simulink model "OnePhInverterCS_17b"  (R2020a)
settings: Solver=ode23tb  StartTime=0.0  StopTime=1  MaxStep=1e-3  RelTol=1e-3
libraries: powerlib x13, powerlib_meascontrol x10
settings Model: Creator=theo  LastModifiedBy=Theodore
settings DebuggingCC: ArithmeticOperatorsInVariantConditions=warning
settings SFSimCC: CustomCodeUndefinedFunction=UseInterfaceOnly

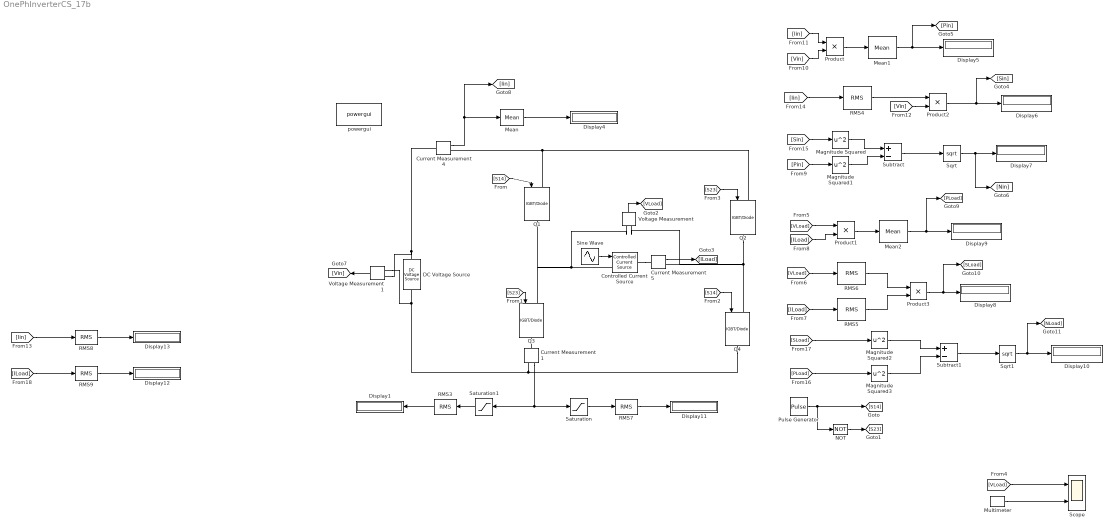
== system OnePhInverterCS_17b ==
  Controlled Current Source : powerlib/Electrical Sources/Controlled Current Source  Initialize=on  Source_Type=AC  Amplitude=10  Phase=0  Frequency=0  Measurements=Current
  Current Measurement1 : powerlib/Measurements/Current Measurement  PhasorSimulation=off  OutputType=Complex  PSBequivalent=0
  Current Measurement4 : powerlib/Measurements/Current Measurement  PhasorSimulation=off  OutputType=Complex  PSBequivalent=0
  Current Measurement5 : powerlib/Measurements/Current Measurement  PhasorSimulation=off  OutputType=Complex  PSBequivalent=0
  DC Voltage Source : powerlib/Electrical Sources/DC Voltage Source  Amplitude=537.97  Measurements=None
  Display{1,4..13} (11 alike) : Display
  Magnitude Squared{,1..3} (4 alike) : Math  Operator=square  SaturateOnIntegerOverflow=on
  Mean : powerlib_meascontrol/Measurements/Mean  Freq=50  Vinit=0  Ts=0
  Mean1 : powerlib_meascontrol/Measurements/Mean  Freq=50  Vinit=0  Ts=0
  Mean2 : powerlib_meascontrol/Measurements/Mean  Freq=50  Vinit=0  Ts=0
  Multimeter : powerlib/Measurements/Multimeter  PhasorSimulation=off  OutputType=Complex  sel=1  L=1  Gain=1  yselected={'Isrc: Controlled Current Source'};  PSBOutputType=1  PSBequivalent=0  AxesSetting=[0,0.1,-100,100]  Display=0  SavedBlockNames=-11
  NOT : Logic  Operator=NOT  IconShape=distinctive  AllPortsSameDT=off  OutDataTypeStr=boolean
  Product{,1..3} (4 alike) : Product
  Pulse Generator : DiscretePulseGenerator  PulseType=Time based  Period=0.02  PulseWidth=50
  Q{1..4} (4 alike) : powerlib/Power Electronics/IGBT//Diode  Ron=1e-3  Rs=1e5  Cs=inf  Measurements=off
  RMS{3..9} (7 alike) : powerlib_meascontrol/Measurements/RMS  TrueRMS=on  Freq=50  RMSInit=120  Ts=0
  Saturation : Saturate  UpperLimit=0  LowerLimit=-100
  Saturation1 : Saturate  UpperLimit=100  LowerLimit=0
  Scope : Scope  NumInputPorts=2
  Sine Wave : Sin  Amplitude=10  Frequency=2*pi*50  Phase=-pi/6  SampleTime=0
  Sqrt : Sqrt  SaturateOnIntegerOverflow=on
  Sqrt1 : Sqrt  SaturateOnIntegerOverflow=on
  Subtract : Sum  Inputs=+-
  Subtract1 : Sum  Inputs=+-
  Voltage Measurement : powerlib/Measurements/Voltage Measurement  PhasorSimulation=off  OutputType=Complex  PSBequivalent=0
  Voltage Measurement1 : powerlib/Measurements/Voltage Measurement  PhasorSimulation=off  OutputType=Complex  PSBequivalent=0
  powergui : powerlib/powergui  Priority=1  SimulationMode=Continuous  SampleTime=50e-6  frequency=60  Iterations=50  frequencyindice=0  Pbase=100e6  ErrMax=1e-4  UnitsV=kV  UnitsW=MW  buscounter=0  FunctionMessages=off  echomessages=off  EnableUseOfTLC=off  CurrentSourceSwitches=off  DisableSnubberDevices=on  DisableRonSwitches=on  DisableVfSwitches=on  DisplayEquations=off  AutomaticDiscreteSolvers=off  SolverType=Tustin/Backward Euler (TBE)  Interpol=off  ExternalGateDelay=off  methode=off  Ts=100  x0status=blocks  SPID=on  SwTol=0  HookPort=off  NonlinearTolerance=1e-4  nMaxIteration=100  ContinueOnMaxIteration=off  RestoreLinks=warning  ResistiveCurrentMeasurement=off  Frange=[0:2:500]  Ylog=off  Xlog=on  ShowGrid=off  save=off  variable=ZData  structure=0  ZoomFFT=off  StartTime=0.0  cycles=1  DisplayStyle=1  fundamental=60  FreqAxis=off  MaxFrequency=1000  frequencyindicesteady=1  RmsSteady=1  display=off
  wires:
  [S14] -> Q1/1
  NOT/1 -> [S23]
  Voltage Measurement/1 -> [VLoad]
  Multimeter/1 -> Scope/2
  [S14] -> Q4/1
  [S23] -> Q3/1
  [VLoad] -> Scope/1
  [S23] -> Q2/1
  Pulse Generator/1 -> NOT/1, [S14]
  Sine Wave/1 -> Controlled Current Source/1
  Current Measurement1/1 -> Saturation1/1, Saturation/1
  Mean/1 -> Display4/1
  [Pin] -> Magnitude Squared1/1
  [Iin] -> Product/1
  Magnitude Squared1/1 -> Subtract/2
  [Iin] -> RMS4/1
  RMS4/1 -> Product2/1
  Sqrt/1 -> [Nin], Display7/1
  [Sin] -> Magnitude Squared/1
  [Vin] -> Product2/2
  [Vin] -> Product/2
  Subtract/1 -> Sqrt/1
  Magnitude Squared/1 -> Subtract/1
  Product2/1 -> [Sin], Display6/1
  Mean1/1 -> [Pin], Display5/1
  Product/1 -> Mean1/1
  Product1/1 -> Mean2/1
  Sqrt1/1 -> [NLoad], Display10/1
  Product3/1 -> [SLoad], Display8/1
  [PLoad] -> Magnitude Squared3/1
  [SLoad] -> Magnitude Squared2/1
  Magnitude Squared2/1 -> Subtract1/1
  Magnitude Squared3/1 -> Subtract1/2
  [ILoad] -> RMS5/1
  RMS6/1 -> Product3/1
  [ILoad] -> Product1/2
  [VLoad] -> Product1/1
  Subtract1/1 -> Sqrt1/1
  Mean2/1 -> [PLoad], Display9/1
  RMS5/1 -> Product3/2
  [VLoad] -> RMS6/1
  Current Measurement4/1 -> [Iin], Mean/1
  Voltage Measurement1/1 -> [Vin]
  Current Measurement5/1 -> [ILoad]
  Saturation/1 -> RMS7/1
  RMS7/1 -> Display11/1
  RMS3/1 -> Display1/1
  Saturation1/1 -> RMS3/1
  RMS8/1 -> Display13/1
  RMS9/1 -> Display12/1
  [ILoad] -> RMS9/1
  [Iin] -> RMS8/1
  connections:
  Q4/RConn1 -- Current Measurement1/RConn1 -- Voltage Measurement1/LConn2 -- DC Voltage Source/LConn1
  Q2/RConn1 -- Voltage Measurement/LConn2 -- Current Measurement5/RConn1 -- Q4/LConn1
  Q1/LConn1 -- Q2/LConn1 -- Current Measurement4/RConn1
  Voltage Measurement/LConn1 -- Controlled Current Source/LConn1 -- Q1/RConn1 -- Q3/LConn1
  Current Measurement1/LConn1 -- Q3/RConn1
  Current Measurement4/LConn1 -- Voltage Measurement1/LConn1 -- DC Voltage Source/RConn1
  Controlled Current Source/RConn1 -- Current Measurement5/LConn1
